simulink model "Furnace"  (R2020a)
settings: Solver=ode15s  StartTime=0  StopTime=12000  FixedStep=0.1  MaxStep=20  RelTol=1e-08  AbsTol=1e-09
undefined symbols (not defined in the file): k, reg
libraries: simulink x9, mpclib x1
(part 3 of 3)

== matlab function Furnace/Plant/Calorific Value/MATLAB Function ==
  data: Fi_fg input; HHV output; T_fg input; cp_fg input; T_amb input; F_aI input; T_aI input; F_aII input; T_aII input
function HHV = CalorificValue(Fi_fg,T_fg,cp_fg,T_amb,F_aI,T_aI,F_aII,T_aII)

HHV = sum(Fi_fg).*cp_fg.*(T_fg-T_amb);%-sum(F_aI).*cp_fg.*(T_aI-T_amb)-F_aII.*cp_fg.*(T_aII-T_amb);

== matlab function Furnace/Grate speed/Input selector2 ==
  data: constant input; signal output; experimental input; controlled input; input_type input
function signal = ChooseSignal(constant, experimental, controlled, input_type)
    switch(input_type)
        case InputType.Experimental
            signal = experimental;
        case InputType.Controlled
            signal = controlled;
        otherwise
            signal = constant;
    end
end

== matlab function Furnace/Controller/Input  selector3 ==
  data: constant input; signal output; experimental input; controlled input; input_type input
function signal = ChooseSignal(constant, experimental, controlled, input_type)
    switch(input_type)
        case InputType.Experimental
            signal = experimental;
        case InputType.Controlled
            signal = controlled;
        otherwise
            signal = constant;
    end
end

== matlab function Furnace/Controller/Input  selector4 ==
  data: constant input; signal output; experimental input; controlled input; input_type input
function signal = ChooseSignal(constant, experimental, controlled, input_type)
    switch(input_type)
        case InputType.Experimental
            signal = experimental;
        case InputType.Controlled
            signal = controlled;
        otherwise
            signal = constant;
    end
end

== matlab function Furnace/Controller/Input  selector5 ==
  data: constant input; signal output; experimental input; controlled input; input_type input
function signal = ChooseSignal(constant, experimental, controlled, input_type)
    switch(input_type)
        case InputType.Experimental
            signal = experimental;
        case InputType.Controlled
            signal = controlled;
        otherwise
            signal = constant;
    end
end

== matlab function Furnace/Controller/Input  selector2 ==
  data: constant input; signal output; experimental input; controlled input; input_type input
function signal = ChooseSignal(constant, experimental, controlled, input_type)
    switch(input_type)
        case InputType.Experimental
            signal = experimental;
        case InputType.Controlled
            signal = controlled;
        otherwise
            signal = constant;
    end
end

== matlab function Furnace/Plant/Grate/Diff_Grate ==
  data: M_w input; dMw_dt_col output; T_w input; M_char input; Fi_w_in input; T_w_in input; F_aI input; T_aI input; Q_rad input; Q_burners input; Q_grate input; v_grate input; L input; Delta_H input; cp_w input; cp_steel input; M_steel_grate input; cp_fg input; Mw_w input; Mw_gas input; p_amb input; T_amb input; k_w input; k_grate input; W input; rho_w input; A_grate input; dTw_dt_col output; dMchar_dt_col output; F_fg_out output; F_flyash output; F_w_ash output; F_char_ash output; t input
function [dMw_dt_col,dTw_dt_col,dMchar_dt_col,F_fg_out,F_flyash,F_w_ash,F_char_ash]= DIFF_Grate(M_w,T_w,M_char,Fi_w_in,T_w_in,F_aI,T_aI,Q_rad,Q_burners,Q_grate,v_grate,L,Delta_H,cp_w,cp_steel,M_steel_grate,cp_fg,Mw_w,Mw_gas,p_amb,T_amb,k_w,k_grate,W,rho_w,A_grate,t)

% This function calculates the mass and energy balance of the furnace. The
% furnace is treated as a one dimensional system, which is discretized in
% 'n_cell'-control volumes, in the direction of movement of the waste on 
% the grate.

%%%%%%%%%%%%%%%%%%%%%%%%%%%%%%%%%%%%%%%%%%%%%%%%%%%%%%%%%%%%%%%%%%%%%%%%%%
% Symbol        Units       Explanation
% INPUTS:
% M_w           [kg]        Mass of waste components in each cell of the furnace
% T_w           [K]         Temperature of waste in each cell ot the furnace
% M_char        [kg]        Mass char in each cell of the furnace
% Fi_w_in       [kg/s]      Waste component mass flows into the furnace (it
%                           enters the first cell of the furnace.
% T_w_in        [K]         Temperature of the waste entering the furnace
% F_aI          [kg/s]      Primary air component mass flows in each zone
%                           (there are 'n_zone'-zones)
% T_aI          [K]         Temperature of primary air (same in every zone)
% Q_rad         [W]         Radiative heat to each cell
% Q_burners     [W]         Toatal heat delivered by auxiliary burners
% Q_grate       [W]         Heat removed by grate cooling (only zones 1-3)
% k              -          Vector of constant parameters
% t             [s]         Time 
%%%%%%%%%%%%%%%%%%%%%%%%%%%%%%%%%%%%%%%%%%%%%%%%%%%%%%%%%%%%%%%%%%%%%%%%%%

%% SOLID WASTE 
T_w         = T_w';
M_char      = M_char';
n_cell      = length(T_w);
nc_w        = length(M_w)./n_cell;
M_w         = reshape(M_w,[nc_w,n_cell]);   % Transform vector M_w into a matrix
Mw_tot      = sum(M_w,1) + M_char;          % Total mass in each zone [kg]

%% GEOMETRTICAL GRID
n_zone      = length(F_aI);
L_zone      = L./n_zone;                    % [m]
L_cell      = L./n_cell;                    % [m]
n           = 50;
x_zone      = linspace(0,L,n*n_zone);
x_cell      = linspace(0,L,n*n_cell);
F_aI_x      = zeros(size(x_zone));
T_aI_x      = zeros(size(x_zone));
Q_grate_x   = zeros(size(x_zone));
if Q_burners > 0
    Q_grate = zeros(5,1);                   % No grate cooling when the burners are on
else 
    Q_grate = [Q_grate; 0; 0];              % There is no grate cooling in zone 4 and 5
end
for i=1:n_zone
    F_aI_x((i-1)*n+1:i*n)   = F_aI(i).*ones(1,n)./L_zone;
    T_aI_x((i-1)*n+1:i*n)   = T_aI.*ones(1,n);
    Q_grate_x((i-1)*n+1:i*n)= Q_grate(i).*ones(1,n)./L_zone;
end
F_aI_dx     = interp1(x_zone,F_aI_x,x_cell);
T_aI_dx     = interp1(x_zone,T_aI_x,x_cell);
Q_grate_dx  = interp1(x_zone,Q_grate_x,x_cell);
F_aI        = zeros(size(T_w));
T_aI        = zeros(size(T_w));
Q_grate     = zeros(size(T_w));

for i = 1:n_cell
    F_aI(1,i)   = trapz(x_cell((i-1)*n+1:i*n),F_aI_dx((i-1)*n+1:i*n));
    T_aI(1,i)   = trapz(x_cell((i-1)*n+1:i*n),F_aI_dx((i-1)*n+1:i*n).*T_aI_dx((i-1)*n+1:i*n))./F_aI(1,i);
    Q_grate(1,i)= trapz(x_cell((i-1)*n+1:i*n),Q_grate_dx((i-1)*n+1:i*n));
end
%% INPUTS 
% Flows and temperature of the waste leaving each cell
Fi_w_out    = zeros(size(M_w));
for i = 1:n_cell
    if t>=(i*L_cell/v_grate)
        Fi_w_out(:,i) = v_grate.*M_w(:,i)./L_cell;
    end
end
T_w_out     = [T_w(:,2:end) T_w(end)];
% Flows and temperature of the waste entering each cell
Fi_w_in     = [Fi_w_in, Fi_w_out(:,1:end-1)];
F_w_in      = sum(Fi_w_in,1);
T_w_in      = [T_w_in, T_w(:,1:end-1)];
% Primary air  
w_aI        = CALC_w_ha(T_amb,90,Mw_gas);
Fi_aI       = zeros(length(w_aI),length(T_w));
for i = 1:n_cell
    Fi_aI(:,i)  = w_aI(:,1).*F_aI(i);
end

%% CONDUCTION TERMS
h_w         = sum(M_w,1)./(rho_w.*W);  % the height of the waste is a function of the mass on the grate
A_w         = W.*h_w;
% Conduction heat through the waste layer
Q_cond_w_in = -k_w.*A_w.*(T_w-T_w_in)./L_cell;
Q_cond_w_out= [Q_cond_w_in(2:end), 0];
Q_cond_w_l = [0 -k_w.*A_w(2:end).*(T_w(2:end)-T_w_in(2:end))./L_cell];
Q_cond_w_r= [Q_cond_w_l(2:end), 0];
% Conduction heat through the metal grate
Q_cond_g_in = -k_grate.*A_grate.*(T_w-T_w_in)./L_cell;
Q_cond_g_out= -k_grate.*A_grate.*(T_w_out-T_w)./L_cell;
Q_cond_g_l = [0 -k_grate.*A_grate.*(T_w(2:end)-T_w_in(2:end))./L_cell];
Q_cond_g_r= [Q_cond_g_l(2:end), 0];
% Total conduction term for each cell 
Q_cond      = Q_cond_w_l - Q_cond_w_r + Q_cond_g_l - Q_cond_g_r;

%% BURNERS
Q_burn      = Q_burners./n_cell.*ones(1,n_cell);

%% REACTION RATES
R_w         = CALC_Rw_Char(M_w,T_w,M_char,Fi_aI,Mw_w,Mw_gas,p_amb);  

%% STATIONARY TOTAL GAS BALANCE
F_fg_out    = Fi_aI + R_w.gas;
F_flyash    = -R_w.waste_cons(end,:);

%% DIFFERENTIAL EQUATIONS
% Solid waste mass balance
F_reac      = R_w.waste_cons;
dMw_dt      = Fi_w_in - Fi_w_out + F_reac;
         
% Char mass balance
F_char_out  = v_grate.*M_char./L_cell;          % [kg/s]
F_char_in   = [0, F_char_out(:,1:end-1)];
F_char_reac = R_w.char + R_w.char_cons;
dMchar_dt   = F_char_in - F_char_out + F_char_reac;       

% Enargy balance
Delta_H_tot = -(R_w.waste_cons(1,:).*Delta_H(1) + ...
                sum(R_w.waste_cons(2:end-1,:)).*Delta_H(2) + ...
                R_w.char_cons.*Delta_H(3) );
dTw_dt      = 1./(cp_w.*Mw_tot +cp_steel.*M_steel_grate./n_cell).*((F_w_in+F_char_in).*cp_w.*(T_w_in-T_w)+F_aI.*cp_fg.*(T_aI-T_w)+...  	% Convective terms
              Delta_H_tot+...                                                                                   % Reaction term
              Q_rad' +...                                                                                       % Radiation term
              Q_cond +...                                                                                       % Conduction term
              Q_burn -...                                                                                       % Burners
              Q_grate);                                                                                         % Grate cooling
% Make outputs into colums
dMw_dt_col   = reshape(dMw_dt,[n_cell*nc_w,1]);
dMchar_dt_col= dMchar_dt';
dTw_dt_col   = dTw_dt';
F_w_ash      = Fi_w_out(end+1-nc_w:end);
F_char_ash   = F_char_out(end);

== matlab function Furnace/Plant/Boiler/Evaporator/Evaporator ==
  data: Fi_fg input; Q_EVA output; T_drum input; T_fg1 input; cp_fg input; epsilon_EVA input; T_fg2 output; eff_HE input
function [Q_EVA, T_fg2] = CALC_Q_EVA(Fi_fg,T_drum,T_fg1,cp_fg,epsilon_EVA,eff_HE)

% This function calculates the heat exchanged in the economizer

F_fg    = sum(Fi_fg);
C_min   = cp_fg.*F_fg;
Q_EVA   = epsilon_EVA.*C_min.*(T_fg1-T_drum);
T_fg2   = T_fg1 - Q_EVA./(cp_fg.*F_fg);
Q_EVA   = Q_EVA.*eff_HE;
